simulink model "Bouncning_ball"  (R2019a)
settings: Solver=VariableStepAuto  StartTime=0.0  StopTime=20.0  RelTol=1e-3
undefined symbols (not defined in the file): g, k, v
settings Model: Creator=aleri934  LastModifiedBy=aleri934

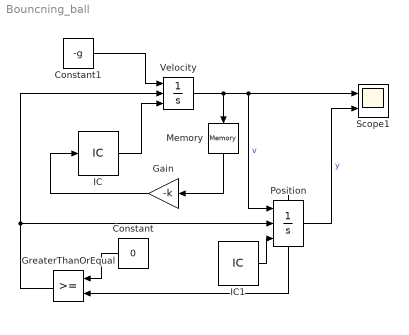
== system Bouncning_ball ==
  Constant : Constant  Value=0
  Constant1 : Constant  Value=-g
  Gain : Gain  Gain=-k
  GreaterThanOrEqual : RelationalOperator  OutDataTypeStr=boolean  RndMeth=Simplest
  IC : InitialCondition  Value=v
  IC1 : InitialCondition  Value=10
  Memory : Memory
  Position : Integrator  ExternalReset=rising  InitialConditionSource=external  InitialCondition=10  ShowStatePort=on
  Scope1 : Scope  NumInputPorts=2
  Velocity : Integrator  ExternalReset=rising  InitialConditionSource=external  InitialCondition=15
  wires:
  Velocity/1 -> Memory/1, Position/1, Scope1/1  "v"
  GreaterThanOrEqual/1 -> Velocity/2, Position/2
  Constant1/1 -> Velocity/1
  Gain/1 -> IC/1
  IC/1 -> Velocity/3
  Memory/1 -> Gain/1
  Constant/1 -> GreaterThanOrEqual/1
  Position/1 -> Scope1/2  "y"
  Position/State -> GreaterThanOrEqual/2
  IC1/1 -> Position/3
